simulink model "CementPlantVer1"  (R2019b)
settings: Solver=ode4  StartTime=0.0  StopTime=inf  FixedStep=0.01  RelTol=1e-3
(part 2 of 2)

== system CementPlantVer1/Clinker Fan 2 ==
  Input Frequence : Inport
  Motor Enable : Inport  Port=2
  Constant : Constant  Value=0
  Divide : Product  Inputs=*/
  Frequency Constant : Constant  Value=50
  Frequency Constant FB : Constant  Value=50
  Motor Transfer Function : TransferFcn  Denominator=[1 3.156 1]
  Output coefficient : Constant  Value=1350
  Product : Product
  Product1 : Product
  Saturation : Saturate  UpperLimit=50  LowerLimit=0
  Switch : Switch  Threshold=1
  Output RPM : Outport
  Output Frequence : Outport  Port=2
  wires:
  Product/1 -> Output RPM/1
  Frequency Constant FB/1 -> Product1/2
  Output coefficient/1 -> Product/1
  Frequency Constant/1 -> Divide/2
  Motor Transfer Function/1 -> Product/2, Product1/1
  Input Frequence/1 -> Divide/1
  Saturation/1 -> Output Frequence/1
  Product1/1 -> Saturation/1
  Divide/1 -> Switch/1
  Switch/1 -> Motor Transfer Function/1
  Motor Enable/1 -> Switch/2
  Constant/1 -> Switch/3

== system CementPlantVer1/Clinker Fan 3 ==
  Input Frequence : Inport
  Motor Enable : Inport  Port=2
  Constant : Constant  Value=0
  Divide : Product  Inputs=*/
  Frequency Constant : Constant  Value=50
  Frequency Constant FB : Constant  Value=50
  Motor Transfer Function : TransferFcn  Denominator=[1 3.156 1]
  Output coefficient : Constant  Value=1350
  Product : Product
  Product1 : Product
  Saturation : Saturate  UpperLimit=50  LowerLimit=0
  Switch : Switch  Threshold=1
  Output RPM : Outport
  Output Frequence : Outport  Port=2
  wires:
  Product/1 -> Output RPM/1
  Frequency Constant FB/1 -> Product1/2
  Output coefficient/1 -> Product/1
  Frequency Constant/1 -> Divide/2
  Motor Transfer Function/1 -> Product/2, Product1/1
  Input Frequence/1 -> Divide/1
  Saturation/1 -> Output Frequence/1
  Product1/1 -> Saturation/1
  Divide/1 -> Switch/1
  Switch/1 -> Motor Transfer Function/1
  Motor Enable/1 -> Switch/2
  Constant/1 -> Switch/3

== system CementPlantVer1/Clinker Fan 4 ==
  Input Frequence : Inport
  Motor Enable : Inport  Port=2
  Constant : Constant  Value=0
  Divide : Product  Inputs=*/
  Frequency Constant : Constant  Value=50
  Frequency Constant FB : Constant  Value=50
  Motor Transfer Function : TransferFcn  Denominator=[1 3.156 1]
  Output coefficient : Constant  Value=1350
  Product : Product
  Product1 : Product
  Saturation : Saturate  UpperLimit=50  LowerLimit=0
  Switch : Switch  Threshold=1
  Output RPM : Outport
  Output Frequence : Outport  Port=2
  wires:
  Product/1 -> Output RPM/1
  Frequency Constant FB/1 -> Product1/2
  Output coefficient/1 -> Product/1
  Frequency Constant/1 -> Divide/2
  Motor Transfer Function/1 -> Product/2, Product1/1
  Input Frequence/1 -> Divide/1
  Saturation/1 -> Output Frequence/1
  Product1/1 -> Saturation/1
  Divide/1 -> Switch/1
  Switch/1 -> Motor Transfer Function/1
  Motor Enable/1 -> Switch/2
  Constant/1 -> Switch/3

== system CementPlantVer1/Clinker In Valve 1 ==
  Opening Percent : Inport
  Enable : Inport  Port=2
  Level of Silo : Inport  Port=3
  Constant : Constant  Value=0
  Delay 1s : TransportDelay
  Divide : Product  Inputs=*/
  Maxium Value : Constant  Value=100
  Output Coefficient : Gain  Gain=OutputGain
  Switch : Switch  Threshold=1
  Switch1 : Switch  Criteria=u2 > Threshold
  Transfer Fnc : TransferFcn  Denominator=[20 1]
  Flow : Outport
  wires:
  Transfer Fnc/1 -> Delay 1s/1
  Enable/1 -> Switch/2
  Constant/1 -> Switch/3, Switch1/3
  Opening Percent/1 -> Divide/1
  Divide/1 -> Switch/1
  Maxium Value/1 -> Divide/2
  Output Coefficient/1 -> Flow/1
  Delay 1s/1 -> Output Coefficient/1
  Switch1/1 -> Transfer Fnc/1
  Switch/1 -> Switch1/1
  Level of Silo/1 -> Switch1/2

== system CementPlantVer1/Clinker In Valve 2 ==
  Opening Percent : Inport
  Enable : Inport  Port=2
  Level of Silo : Inport  Port=3
  Constant : Constant  Value=0
  Delay 1s : TransportDelay
  Divide : Product  Inputs=*/
  Maxium Value : Constant  Value=100
  Output Coefficient : Gain  Gain=OutputGain
  Switch : Switch  Threshold=1
  Switch1 : Switch  Criteria=u2 > Threshold
  Transfer Fnc : TransferFcn  Denominator=[20 1]
  Flow : Outport
  wires:
  Transfer Fnc/1 -> Delay 1s/1
  Enable/1 -> Switch/2
  Constant/1 -> Switch/3, Switch1/3
  Opening Percent/1 -> Divide/1
  Divide/1 -> Switch/1
  Maxium Value/1 -> Divide/2
  Output Coefficient/1 -> Flow/1
  Delay 1s/1 -> Output Coefficient/1
  Switch1/1 -> Transfer Fnc/1
  Switch/1 -> Switch1/1
  Level of Silo/1 -> Switch1/2

== system CementPlantVer1/Clinker PreHeater System ==
  RPM In 1 : Inport
  RPM In 2 : Inport  Port=2
  Flow In : Inport  Port=3
  Enable 10 : Constant
  Enable 8 : Constant
  Power supplied to PreHeater 1 : Subsystem
  Power supplied to PreHeater 2 : Subsystem
  PreHeater Flow Transfer Fnc : TransferFcn  Denominator=[0.5 1]
  PreHeater System : Subsystem
  Sum4 : Sum  Inputs=|++
  Temperature : Outport
  Flow out : Outport  Port=2
  wires:
  Enable 8/1 -> Power supplied to PreHeater 1/2(Enable)
  Enable 10/1 -> Power supplied to PreHeater 2/2(Enable)
  Power supplied to PreHeater 1/1(Power Percent) -> Sum4/1
  Sum4/1 -> PreHeater System/1(Power Percent)
  PreHeater System/1(Temperature) -> Temperature/1
  RPM In 2/1 -> Power supplied to PreHeater 2/1(RPM)
  Power supplied to PreHeater 2/1(Power Percent) -> Sum4/2
  RPM In 1/1 -> Power supplied to PreHeater 1/1(RPM)
  Flow In/1 -> PreHeater Flow Transfer Fnc/1
  PreHeater Flow Transfer Fnc/1 -> Flow out/1

== system CementPlantVer1/Clinker Rotary Kiln ==
  RPM In 1 : Inport
  RPM In 2 : Inport  Port=2
  RPM In 3 : Inport  Port=3
  Flow In : Inport  Port=4
  Rotary Kiln Frequence : Inport  Port=5
  Clinker : Subsystem
  Enable 2 : Constant
  Enable 4 : Constant
  Enable 6 : Constant
  Power supplied to Clinker 1 : Subsystem
  Power supplied to Clinker 2 : Subsystem
  Power supplied to Clinker 3 : Subsystem
  Rotary Kiln Motor : Subsystem
  Sum : Sum  Inputs=3
  Temperature : Outport
  Flow Out : Outport  Port=2
  Rotary Kiln RPM : Outport  Port=3
  Rotary Kiln Frequence FB : Outport  Port=4
  wires:
  Sum/1 -> Clinker/1(Power Percent)
  Enable 4/1 -> Power supplied to Clinker 2/2(Enable)
  Enable 2/1 -> Power supplied to Clinker 1/2(Enable)
  Clinker/1(Temperature) -> Temperature/1
  RPM In 3/1 -> Power supplied to Clinker 3/1(RPM)
  Power supplied to Clinker 1/1(Power Percent) -> Sum/1
  Power supplied to Clinker 2/1(Power Percent) -> Sum/2
  Power supplied to Clinker 3/1(Power Percent) -> Sum/3
  Enable 6/1 -> Power supplied to Clinker 3/2(Enable)
  RPM In 2/1 -> Power supplied to Clinker 2/1(RPM)
  RPM In 1/1 -> Power supplied to Clinker 1/1(RPM)
  Flow In/1 -> Rotary Kiln Motor/1(Flow In)
  Rotary Kiln Frequence/1 -> Rotary Kiln Motor/2(Frequence In)
  Rotary Kiln Motor/1(Flow out) -> Flow Out/1
  Rotary Kiln Motor/2(RPM out) -> Rotary Kiln RPM/1
  Rotary Kiln Motor/3(Frequence FB) -> Rotary Kiln Frequence FB/1

== system CementPlantVer1/Clinker Silo 1 ==
  Qin : Inport
  Qout : Inport  Port=2
  A : Gain  Gain=1/(3.14*3*3)
  Convert h to s : Constant  Value=3600
  Density of Clay : Constant  Value=DensityOfMaterial
  Divide : Product  Inputs=*/
  Divide1 : Product  Inputs=*/
  High Operator : RelationalOperator  OutDataTypeStr=boolean  RndMeth=Simplest
  High Level Set (m) : Constant  Value=HighLevelSet
  Low Operator : RelationalOperator  Operator=<=  OutDataTypeStr=boolean  RndMeth=Simplest
  Low Level Set (m) : Constant  Value=LowLevelSet
  Output Coefficient : Gain  Gain=OutputGain
  Saturation Limit : Saturate  UpperLimit=20  LowerLimit=0
  Sum1 : Sum  Inputs=|+-
  Transfer Fnc of Silo : TransferFcn  Denominator=[1 0]
  Level : Outport
  High : Outport  Port=2
  Low : Outport  Port=3
  wires:
  A/1 -> Output Coefficient/1
  Low Operator/1 -> Low/1
  High Level Set (m)/1 -> High Operator/2
  Low Level Set (m)/1 -> Low Operator/2
  Density of Clay/1 -> Divide/2
  Output Coefficient/1 -> Saturation Limit/1
  Convert h to s/1 -> Divide1/2
  Transfer Fnc of Silo/1 -> A/1
  Divide1/1 -> Transfer Fnc of Silo/1
  High Operator/1 -> High/1
  Saturation Limit/1 -> Level/1, Low Operator/1, High Operator/1
  Divide/1 -> Divide1/1
  Sum1/1 -> Divide/1
  Qin/1 -> Sum1/1
  Qout/1 -> Sum1/2

== system CementPlantVer1/Clinker Silo 2 ==
  Qin : Inport
  Qout : Inport  Port=2
  A : Gain  Gain=1/(3.14*3*3)
  Convert h to s : Constant  Value=3600
  Density of Clay : Constant  Value=DensityOfMaterial
  Divide : Product  Inputs=*/
  Divide1 : Product  Inputs=*/
  High Operator : RelationalOperator  OutDataTypeStr=boolean  RndMeth=Simplest
  High Level Set (m) : Constant  Value=HighLevelSet
  Low Operator : RelationalOperator  Operator=<=  OutDataTypeStr=boolean  RndMeth=Simplest
  Low Level Set (m) : Constant  Value=LowLevelSet
  Output Coefficient : Gain  Gain=OutputGain
  Saturation Limit : Saturate  UpperLimit=20  LowerLimit=0
  Sum1 : Sum  Inputs=|+-
  Transfer Fnc of Silo : TransferFcn  Denominator=[1 0]
  Level : Outport
  High : Outport  Port=2
  Low : Outport  Port=3
  wires:
  A/1 -> Output Coefficient/1
  Low Operator/1 -> Low/1
  High Level Set (m)/1 -> High Operator/2
  Low Level Set (m)/1 -> Low Operator/2
  Density of Clay/1 -> Divide/2
  Output Coefficient/1 -> Saturation Limit/1
  Convert h to s/1 -> Divide1/2
  Transfer Fnc of Silo/1 -> A/1
  Divide1/1 -> Transfer Fnc of Silo/1
  High Operator/1 -> High/1
  Saturation Limit/1 -> Level/1, Low Operator/1, High Operator/1
  Divide/1 -> Divide1/1
  Sum1/1 -> Divide/1
  Qin/1 -> Sum1/1
  Qout/1 -> Sum1/2

== system CementPlantVer1/CoalMill Fan 1 ==
  Input Frequence : Inport
  Motor Enable : Inport  Port=2
  Constant : Constant  Value=0
  Divide : Product  Inputs=*/
  Frequency Constant : Constant  Value=50
  Frequency Constant FB : Constant  Value=50
  Motor Transfer Function : TransferFcn  Denominator=[1 3.156 1]
  Output coefficient : Constant  Value=1350
  Product : Product
  Product1 : Product
  Saturation : Saturate  UpperLimit=50  LowerLimit=0
  Switch : Switch  Threshold=1
  Output RPM : Outport
  Output Frequence : Outport  Port=2
  wires:
  Product/1 -> Output RPM/1
  Frequency Constant FB/1 -> Product1/2
  Output coefficient/1 -> Product/1
  Frequency Constant/1 -> Divide/2
  Motor Transfer Function/1 -> Product/2, Product1/1
  Input Frequence/1 -> Divide/1
  Saturation/1 -> Output Frequence/1
  Product1/1 -> Saturation/1
  Divide/1 -> Switch/1
  Switch/1 -> Motor Transfer Function/1
  Motor Enable/1 -> Switch/2
  Constant/1 -> Switch/3

== system CementPlantVer1/CoalMill Pump 1 ==
  Input Frequence : Inport
  Motor Enable : Inport  Port=2
  Constant : Constant  Value=0
  Divide : Product  Inputs=*/
  Frequency Constant : Constant  Value=50
  Frequency Constant FB : Constant  Value=50
  Motor Transfer Function : TransferFcn  Denominator=[1 1.1 1]
  Output coefficient : Constant  Value=1350
  Product : Product
  Product1 : Product
  Saturation : Saturate  UpperLimit=50  LowerLimit=0
  Switch : Switch  Threshold=1
  Output RPM : Outport
  Output Frequence : Outport  Port=2
  wires:
  Product/1 -> Output RPM/1
  Frequency Constant FB/1 -> Product1/2
  Output coefficient/1 -> Product/1
  Frequency Constant/1 -> Divide/2
  Motor Transfer Function/1 -> Product/2, Product1/1
  Input Frequence/1 -> Divide/1
  Saturation/1 -> Output Frequence/1
  Product1/1 -> Saturation/1
  Divide/1 -> Switch/1
  Switch/1 -> Motor Transfer Function/1
  Motor Enable/1 -> Switch/2
  Constant/1 -> Switch/3

== system CementPlantVer1/CoalMill Pump 2 ==
  Input Frequence : Inport
  Motor Enable : Inport  Port=2
  Constant : Constant  Value=0
  Divide : Product  Inputs=*/
  Frequency Constant : Constant  Value=50
  Frequency Constant FB : Constant  Value=50
  Motor Transfer Function : TransferFcn  Denominator=[1 1.1 1]
  Output coefficient : Constant  Value=1350
  Product : Product
  Product1 : Product
  Saturation : Saturate  UpperLimit=50  LowerLimit=0
  Switch : Switch  Threshold=1
  Output RPM : Outport
  Output Frequence : Outport  Port=2
  wires:
  Product/1 -> Output RPM/1
  Frequency Constant FB/1 -> Product1/2
  Output coefficient/1 -> Product/1
  Frequency Constant/1 -> Divide/2
  Motor Transfer Function/1 -> Product/2, Product1/1
  Input Frequence/1 -> Divide/1
  Saturation/1 -> Output Frequence/1
  Product1/1 -> Saturation/1
  Divide/1 -> Switch/1
  Switch/1 -> Motor Transfer Function/1
  Motor Enable/1 -> Switch/2
  Constant/1 -> Switch/3

== system CementPlantVer1/CoalMill Pump 3 ==
  Input Frequence : Inport
  Motor Enable : Inport  Port=2
  Constant : Constant  Value=0
  Divide : Product  Inputs=*/
  Frequency Constant : Constant  Value=50
  Frequency Constant FB : Constant  Value=50
  Motor Transfer Function : TransferFcn  Denominator=[1 1.1 1]
  Output coefficient : Constant  Value=1350
  Product : Product
  Product1 : Product
  Saturation : Saturate  UpperLimit=50  LowerLimit=0
  Switch : Switch  Threshold=1
  Output RPM : Outport
  Output Frequence : Outport  Port=2
  wires:
  Product/1 -> Output RPM/1
  Frequency Constant FB/1 -> Product1/2
  Output coefficient/1 -> Product/1
  Frequency Constant/1 -> Divide/2
  Motor Transfer Function/1 -> Product/2, Product1/1
  Input Frequence/1 -> Divide/1
  Saturation/1 -> Output Frequence/1
  Product1/1 -> Saturation/1
  Divide/1 -> Switch/1
  Switch/1 -> Motor Transfer Function/1
  Motor Enable/1 -> Switch/2
  Constant/1 -> Switch/3

== system CementPlantVer1/CoalMill Pump 4 ==
  Input Frequence : Inport
  Motor Enable : Inport  Port=2
  Constant : Constant  Value=0
  Divide : Product  Inputs=*/
  Frequency Constant : Constant  Value=50
  Frequency Constant FB : Constant  Value=50
  Motor Transfer Function : TransferFcn  Denominator=[1 1.1 1]
  Output coefficient : Constant  Value=1350
  Product : Product
  Product1 : Product
  Saturation : Saturate  UpperLimit=50  LowerLimit=0
  Switch : Switch  Threshold=1
  Output RPM : Outport
  Output Frequence : Outport  Port=2
  wires:
  Product/1 -> Output RPM/1
  Frequency Constant FB/1 -> Product1/2
  Output coefficient/1 -> Product/1
  Frequency Constant/1 -> Divide/2
  Motor Transfer Function/1 -> Product/2, Product1/1
  Input Frequence/1 -> Divide/1
  Saturation/1 -> Output Frequence/1
  Product1/1 -> Saturation/1
  Divide/1 -> Switch/1
  Switch/1 -> Motor Transfer Function/1
  Motor Enable/1 -> Switch/2
  Constant/1 -> Switch/3

== system CementPlantVer1/Gypsum Silo ==
  Qin : Inport
  Qout : Inport  Port=2
  A : Gain  Gain=1/(3.14*3*3)
  Convert h to s : Constant  Value=3600
  Density of Clay : Constant  Value=DensityOfMaterial
  Divide : Product  Inputs=*/
  Divide1 : Product  Inputs=*/
  High Operator : RelationalOperator  OutDataTypeStr=boolean  RndMeth=Simplest
  High Level Set (m) : Constant  Value=HighLevelSet
  Low Operator : RelationalOperator  Operator=<=  OutDataTypeStr=boolean  RndMeth=Simplest
  Low Level Set (m) : Constant  Value=LowLevelSet
  Output Coefficient : Gain  Gain=OutputGain
  Saturation Limit : Saturate  UpperLimit=20  LowerLimit=0
  Sum1 : Sum  Inputs=|+-
  Transfer Fnc of Silo : TransferFcn  Denominator=[1 0]
  Level : Outport
  High : Outport  Port=2
  Low : Outport  Port=3
  wires:
  A/1 -> Output Coefficient/1
  Low Operator/1 -> Low/1
  High Level Set (m)/1 -> High Operator/2
  Low Level Set (m)/1 -> Low Operator/2
  Density of Clay/1 -> Divide/2
  Output Coefficient/1 -> Saturation Limit/1
  Convert h to s/1 -> Divide1/2
  Transfer Fnc of Silo/1 -> A/1
  Divide1/1 -> Transfer Fnc of Silo/1
  High Operator/1 -> High/1
  Saturation Limit/1 -> Level/1, Low Operator/1, High Operator/1
  Divide/1 -> Divide1/1
  Sum1/1 -> Divide/1
  Qin/1 -> Sum1/1
  Qout/1 -> Sum1/2

== system CementPlantVer1/Iron Silo ==
  Qin : Inport
  Qout : Inport  Port=2
  A : Gain  Gain=1/(3.14*3*3)
  Convert h to s : Constant  Value=3600
  Density of Clay : Constant  Value=DensityOfMaterial
  Divide : Product  Inputs=*/
  Divide1 : Product  Inputs=*/
  High Operator : RelationalOperator  OutDataTypeStr=boolean  RndMeth=Simplest
  High Level Set (m) : Constant  Value=HighLevelSet
  Low Operator : RelationalOperator  Operator=<=  OutDataTypeStr=boolean  RndMeth=Simplest
  Low Level Set (m) : Constant  Value=LowLevelSet
  Output Coefficient : Gain  Gain=OutputGain
  Saturation Limit : Saturate  UpperLimit=20  LowerLimit=0
  Sum1 : Sum  Inputs=|+-
  Transfer Fnc of Silo : TransferFcn  Denominator=[1 0]
  Level : Outport
  High : Outport  Port=2
  Low : Outport  Port=3
  wires:
  A/1 -> Output Coefficient/1
  Low Operator/1 -> Low/1
  High Level Set (m)/1 -> High Operator/2
  Low Level Set (m)/1 -> Low Operator/2
  Density of Clay/1 -> Divide/2
  Output Coefficient/1 -> Saturation Limit/1
  Convert h to s/1 -> Divide1/2
  Transfer Fnc of Silo/1 -> A/1
  Divide1/1 -> Transfer Fnc of Silo/1
  High Operator/1 -> High/1
  Saturation Limit/1 -> Level/1, Low Operator/1, High Operator/1
  Divide/1 -> Divide1/1
  Sum1/1 -> Divide/1
  Qin/1 -> Sum1/1
  Qout/1 -> Sum1/2

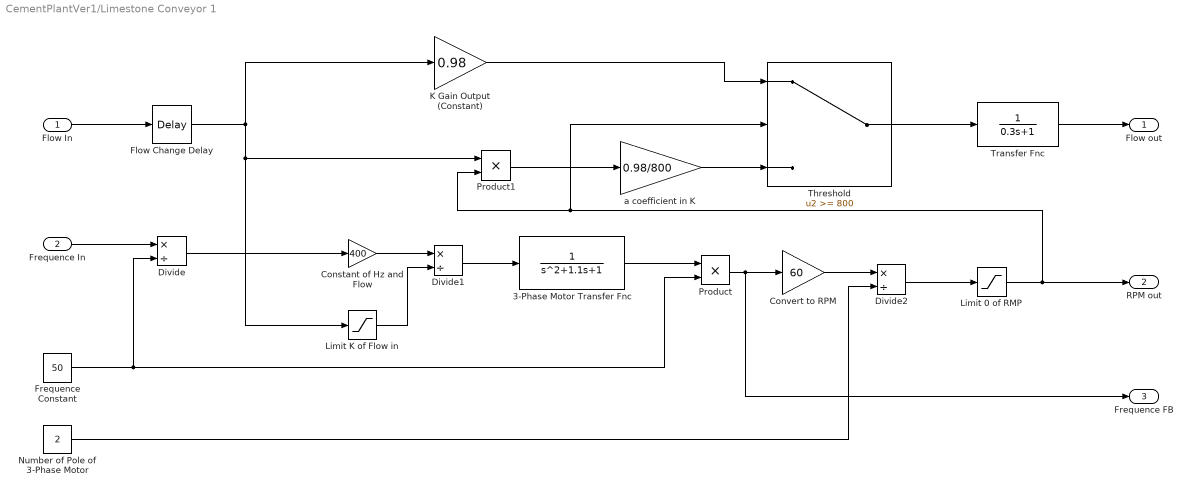
== system CementPlantVer1/Limestone Conveyor 1 ==
  Flow In : Inport
  Frequence In : Inport  Port=2
  3-Phase Motor Transfer Fnc : TransferFcn  Denominator=[1 1.1 1]
  Constant of Hz and Flow : Gain  Gain=400
  Convert to RPM : Gain  Gain=60
  Divide : Product  Inputs=*/
  Divide1 : Product  Inputs=*/
  Divide2 : Product  Inputs=*/
  Flow Change Delay : TransportDelay  DelayTime=0.5
  Frequence Constant : Constant  Value=50
  K Gain Output (Constant) : Gain  Gain=0.98
  Limit 0 of RMP : Saturate  UpperLimit=inf  LowerLimit=0
  Limit K of Flow in : Saturate  UpperLimit=inf  LowerLimit=400
  Number of Pole of 3-Phase Motor : Constant  Value=2
  Product : Product
  Product1 : Product
  Threshold : Switch  Threshold=800
  Transfer Fnc : TransferFcn  Denominator=[0.3 1]
  a coefficient in K : Gain  Gain=0.98/800
  Flow out : Outport
  RPM out : Outport  Port=2
  Frequence FB : Outport  Port=3
  wires:
  Constant of Hz and Flow/1 -> Divide1/1
  Limit K of Flow in/1 -> Divide1/2
  Divide1/1 -> 3-Phase Motor Transfer Fnc/1
  Limit 0 of RMP/1 -> RPM out/1, Threshold/2, Product1/2
  Flow In/1 -> Flow Change Delay/1
  Flow Change Delay/1 -> Product1/1, Limit K of Flow in/1, K Gain Output (Constant)/1
  K Gain Output (Constant)/1 -> Threshold/1
  Frequence In/1 -> Divide/1
  Divide/1 -> Constant of Hz and Flow/1
  Frequence Constant/1 -> Product/2, Divide/2
  3-Phase Motor Transfer Fnc/1 -> Product/1
  Product/1 -> Frequence FB/1, Convert to RPM/1
  Convert to RPM/1 -> Divide2/1
  Divide2/1 -> Limit 0 of RMP/1
  Number of Pole of 3-Phase Motor/1 -> Divide2/2
  Threshold/1 -> Transfer Fnc/1
  Transfer Fnc/1 -> Flow out/1
  Product1/1 -> a coefficient in K/1
  a coefficient in K/1 -> Threshold/3

== system CementPlantVer1/Limestone Conveyor 2 ==
  Flow In : Inport
  Frequence In : Inport  Port=2
  3-Phase Motor Transfer Fnc : TransferFcn  Denominator=[1 1.1 1]
  Constant of Hz and Flow : Gain  Gain=400
  Convert to RPM : Gain  Gain=60
  Divide : Product  Inputs=*/
  Divide1 : Product  Inputs=*/
  Divide2 : Product  Inputs=*/
  Flow Change Delay : TransportDelay  DelayTime=0.5
  Frequence Constant : Constant  Value=50
  K Gain Output (Constant) : Gain  Gain=0.98
  Limit 0 of RMP : Saturate  UpperLimit=inf  LowerLimit=0
  Limit K of Flow in : Saturate  UpperLimit=inf  LowerLimit=400
  Number of Pole of 3-Phase Motor : Constant  Value=2
  Product : Product
  Product1 : Product
  Threshold : Switch  Threshold=800
  Transfer Fnc : TransferFcn  Denominator=[0.3 1]
  a coefficient in K : Gain  Gain=0.98/800
  Flow out : Outport
  RPM out : Outport  Port=2
  Frequence FB : Outport  Port=3
  wires:
  Constant of Hz and Flow/1 -> Divide1/1
  Limit K of Flow in/1 -> Divide1/2
  Divide1/1 -> 3-Phase Motor Transfer Fnc/1
  Limit 0 of RMP/1 -> RPM out/1, Threshold/2, Product1/2
  Flow In/1 -> Flow Change Delay/1
  Flow Change Delay/1 -> Product1/1, Limit K of Flow in/1, K Gain Output (Constant)/1
  K Gain Output (Constant)/1 -> Threshold/1
  Frequence In/1 -> Divide/1
  Divide/1 -> Constant of Hz and Flow/1
  Frequence Constant/1 -> Product/2, Divide/2
  3-Phase Motor Transfer Fnc/1 -> Product/1
  Product/1 -> Frequence FB/1, Convert to RPM/1
  Convert to RPM/1 -> Divide2/1
  Divide2/1 -> Limit 0 of RMP/1
  Number of Pole of 3-Phase Motor/1 -> Divide2/2
  Threshold/1 -> Transfer Fnc/1
  Transfer Fnc/1 -> Flow out/1
  Product1/1 -> a coefficient in K/1
  a coefficient in K/1 -> Threshold/3

== system CementPlantVer1/Limestone Conveyor 3 ==
  Flow In : Inport
  Frequence In : Inport  Port=2
  3-Phase Motor Transfer Fnc : TransferFcn  Denominator=[1 1.1 1]
  Constant of Hz and Flow : Gain  Gain=400
  Convert to RPM : Gain  Gain=60
  Divide : Product  Inputs=*/
  Divide1 : Product  Inputs=*/
  Divide2 : Product  Inputs=*/
  Flow Change Delay : TransportDelay  DelayTime=0.5
  Frequence Constant : Constant  Value=50
  K Gain Output (Constant) : Gain  Gain=0.98
  Limit 0 of RMP : Saturate  UpperLimit=inf  LowerLimit=0
  Limit K of Flow in : Saturate  UpperLimit=inf  LowerLimit=400
  Number of Pole of 3-Phase Motor : Constant  Value=2
  Product : Product
  Product1 : Product
  Threshold : Switch  Threshold=800
  Transfer Fnc : TransferFcn  Denominator=[0.3 1]
  a coefficient in K : Gain  Gain=0.98/800
  Flow out : Outport
  RPM out : Outport  Port=2
  Frequence FB : Outport  Port=3
  wires:
  Constant of Hz and Flow/1 -> Divide1/1
  Limit K of Flow in/1 -> Divide1/2
  Divide1/1 -> 3-Phase Motor Transfer Fnc/1
  Limit 0 of RMP/1 -> RPM out/1, Threshold/2, Product1/2
  Flow In/1 -> Flow Change Delay/1
  Flow Change Delay/1 -> Product1/1, Limit K of Flow in/1, K Gain Output (Constant)/1
  K Gain Output (Constant)/1 -> Threshold/1
  Frequence In/1 -> Divide/1
  Divide/1 -> Constant of Hz and Flow/1
  Frequence Constant/1 -> Product/2, Divide/2
  3-Phase Motor Transfer Fnc/1 -> Product/1
  Product/1 -> Frequence FB/1, Convert to RPM/1
  Convert to RPM/1 -> Divide2/1
  Divide2/1 -> Limit 0 of RMP/1
  Number of Pole of 3-Phase Motor/1 -> Divide2/2
  Threshold/1 -> Transfer Fnc/1
  Transfer Fnc/1 -> Flow out/1
  Product1/1 -> a coefficient in K/1
  a coefficient in K/1 -> Threshold/3

== system CementPlantVer1/Limestone Crusher 1 ==
  Flow In : Inport
  Frequence In : Inport  Port=2
  3-Phase Motor Transfer Fnc : TransferFcn  Denominator=[1 2.5 1]
  Constant of Hz and Flow : Gain  Gain=400
  Convert to RPM : Gain  Gain=60
  Divide : Product  Inputs=*/
  Divide1 : Product  Inputs=*/
  Divide2 : Product  Inputs=*/
  Flow Change Delay : TransportDelay  DelayTime=0.5
  Frequence Constant : Constant  Value=50
  K Gain Output (Constant) : Gain
  Limit 0 of RMP : Saturate  UpperLimit=inf  LowerLimit=0
  Limit K of Flow in : Saturate  UpperLimit=inf  LowerLimit=400
  Number of Pole of 3-Phase Motor : Constant  Value=2
  Product : Product
  Product1 : Product
  Threshold : Switch  Threshold=800
  Transfer Fnc : TransferFcn  Denominator=[0.1 1]
  a coefficient in K : Gain  Gain=1/800
  Flow out : Outport
  Frequence FB : Outport  Port=2
  wires:
  Constant of Hz and Flow/1 -> Divide1/1
  Limit K of Flow in/1 -> Divide1/2
  Divide1/1 -> 3-Phase Motor Transfer Fnc/1
  Limit 0 of RMP/1 -> Threshold/2, Product1/2
  Flow In/1 -> Flow Change Delay/1
  Flow Change Delay/1 -> Product1/1, Limit K of Flow in/1, K Gain Output (Constant)/1
  K Gain Output (Constant)/1 -> Threshold/1
  Frequence In/1 -> Divide/1
  Divide/1 -> Constant of Hz and Flow/1
  Frequence Constant/1 -> Product/2, Divide/2
  3-Phase Motor Transfer Fnc/1 -> Product/1
  Product/1 -> Frequence FB/1, Convert to RPM/1
  Convert to RPM/1 -> Divide2/1
  Divide2/1 -> Limit 0 of RMP/1
  Number of Pole of 3-Phase Motor/1 -> Divide2/2
  Threshold/1 -> Transfer Fnc/1
  Transfer Fnc/1 -> Flow out/1
  Product1/1 -> a coefficient in K/1
  a coefficient in K/1 -> Threshold/3

== system CementPlantVer1/Limestone Crusher 2 ==
  Flow In : Inport
  Frequence In : Inport  Port=2
  3-Phase Motor Transfer Fnc : TransferFcn  Denominator=[1 2.5 1]
  Constant of Hz and Flow : Gain  Gain=400
  Convert to RPM : Gain  Gain=60
  Divide : Product  Inputs=*/
  Divide1 : Product  Inputs=*/
  Divide2 : Product  Inputs=*/
  Flow Change Delay : TransportDelay  DelayTime=0.5
  Frequence Constant : Constant  Value=50
  K Gain Output (Constant) : Gain
  Limit 0 of RMP : Saturate  UpperLimit=inf  LowerLimit=0
  Limit K of Flow in : Saturate  UpperLimit=inf  LowerLimit=400
  Number of Pole of 3-Phase Motor : Constant  Value=2
  Product : Product
  Product1 : Product
  Threshold : Switch  Threshold=800
  Transfer Fnc : TransferFcn  Denominator=[0.1 1]
  a coefficient in K : Gain  Gain=1/800
  Flow out : Outport
  Frequence FB : Outport  Port=2
  wires:
  Constant of Hz and Flow/1 -> Divide1/1
  Limit K of Flow in/1 -> Divide1/2
  Divide1/1 -> 3-Phase Motor Transfer Fnc/1
  Limit 0 of RMP/1 -> Threshold/2, Product1/2
  Flow In/1 -> Flow Change Delay/1
  Flow Change Delay/1 -> Product1/1, Limit K of Flow in/1, K Gain Output (Constant)/1
  K Gain Output (Constant)/1 -> Threshold/1
  Frequence In/1 -> Divide/1
  Divide/1 -> Constant of Hz and Flow/1
  Frequence Constant/1 -> Product/2, Divide/2
  3-Phase Motor Transfer Fnc/1 -> Product/1
  Product/1 -> Frequence FB/1, Convert to RPM/1
  Convert to RPM/1 -> Divide2/1
  Divide2/1 -> Limit 0 of RMP/1
  Number of Pole of 3-Phase Motor/1 -> Divide2/2
  Threshold/1 -> Transfer Fnc/1
  Transfer Fnc/1 -> Flow out/1
  Product1/1 -> a coefficient in K/1
  a coefficient in K/1 -> Threshold/3

== system CementPlantVer1/Limestone Storage ==
  Qin : Inport
  Qout : Inport  Port=2
  A : Gain  Gain=1/(3.14*3*3)
  Convert h to s : Constant  Value=3600
  Density of Clay : Constant  Value=DensityOfMaterial
  Divide : Product  Inputs=*/
  Divide1 : Product  Inputs=*/
  High Operator : RelationalOperator  OutDataTypeStr=boolean  RndMeth=Simplest
  High Level Set (m) : Constant  Value=HighLevelSet
  Low Operator : RelationalOperator  Operator=<=  OutDataTypeStr=boolean  RndMeth=Simplest
  Low Level Set (m) : Constant  Value=LowLevelSet
  Output Coefficient : Gain  Gain=OutputGain
  Saturation Limit : Saturate  UpperLimit=20  LowerLimit=0
  Sum1 : Sum  Inputs=|+-
  Transfer Fnc of Silo : TransferFcn  Denominator=[1 0]
  Level : Outport
  High : Outport  Port=2
  Low : Outport  Port=3
  wires:
  A/1 -> Output Coefficient/1
  Low Operator/1 -> Low/1
  High Level Set (m)/1 -> High Operator/2
  Low Level Set (m)/1 -> Low Operator/2
  Density of Clay/1 -> Divide/2
  Output Coefficient/1 -> Saturation Limit/1
  Convert h to s/1 -> Divide1/2
  Transfer Fnc of Silo/1 -> A/1
  Divide1/1 -> Transfer Fnc of Silo/1
  High Operator/1 -> High/1
  Saturation Limit/1 -> Level/1, Low Operator/1, High Operator/1
  Divide/1 -> Divide1/1
  Sum1/1 -> Divide/1
  Qin/1 -> Sum1/1
  Qout/1 -> Sum1/2

== system CementPlantVer1/Limestone Valve 1 ==
  Opening Percent : Inport
  Enable : Inport  Port=2
  Level of Silo : Inport  Port=3
  Constant : Constant  Value=0
  Delay 1s : TransportDelay
  Divide : Product  Inputs=*/
  Maxium Value : Constant  Value=100
  Output Coefficient : Gain  Gain=OutputGain
  Switch : Switch  Threshold=1
  Switch1 : Switch  Criteria=u2 > Threshold
  Transfer Fnc : TransferFcn  Denominator=[20 1]
  Flow : Outport
  wires:
  Transfer Fnc/1 -> Delay 1s/1
  Enable/1 -> Switch/2
  Constant/1 -> Switch/3, Switch1/3
  Opening Percent/1 -> Divide/1
  Divide/1 -> Switch/1
  Maxium Value/1 -> Divide/2
  Output Coefficient/1 -> Flow/1
  Delay 1s/1 -> Output Coefficient/1
  Switch1/1 -> Transfer Fnc/1
  Switch/1 -> Switch1/1
  Level of Silo/1 -> Switch1/2

== system CementPlantVer1/RawMill Conveyor 1 ==
  Input Frequence : Inport
  Enable : Inport  Port=2
  3-Phase Motor Transfer Fnc : TransferFcn  Denominator=[1 1 1]
  Constant : Constant  Value=0
  Divide : Product  Inputs=*/
  Frequence Coefficient : Gain  Gain=50
  Maxium Value : Constant  Value=50
  Output Coefficient : Gain  Gain=OutputGain
  Switch : Switch  Threshold=1
  Flow : Outport
  FeedBack Frequence : Outport  Port=2
  wires:
  3-Phase Motor Transfer Fnc/1 -> Frequence Coefficient/1, Output Coefficient/1
  Output Coefficient/1 -> Flow/1
  Switch/1 -> 3-Phase Motor Transfer Fnc/1
  Enable/1 -> Switch/2
  Constant/1 -> Switch/3
  Input Frequence/1 -> Divide/1
  Divide/1 -> Switch/1
  Maxium Value/1 -> Divide/2
  Frequence Coefficient/1 -> FeedBack Frequence/1

== system CementPlantVer1/RawMill Conveyor 2 ==
  Input Frequence : Inport
  Enable : Inport  Port=2
  3-Phase Motor Transfer Fnc : TransferFcn  Denominator=[1 1 1]
  Constant : Constant  Value=0
  Divide : Product  Inputs=*/
  Frequence Coefficient : Gain  Gain=50
  Maxium Value : Constant  Value=50
  Output Coefficient : Gain  Gain=OutputGain
  Switch : Switch  Threshold=1
  Flow : Outport
  FeedBack Frequence : Outport  Port=2
  wires:
  3-Phase Motor Transfer Fnc/1 -> Frequence Coefficient/1, Output Coefficient/1
  Output Coefficient/1 -> Flow/1
  Switch/1 -> 3-Phase Motor Transfer Fnc/1
  Enable/1 -> Switch/2
  Constant/1 -> Switch/3
  Input Frequence/1 -> Divide/1
  Divide/1 -> Switch/1
  Maxium Value/1 -> Divide/2
  Frequence Coefficient/1 -> FeedBack Frequence/1

== system CementPlantVer1/RawMill Conveyor 3 ==
  Flow In : Inport
  Frequence In : Inport  Port=2
  3-Phase Motor Transfer Fnc : TransferFcn  Denominator=[1 1.1 1]
  Constant of Hz and Flow : Gain  Gain=400
  Convert to RPM : Gain  Gain=60
  Divide : Product  Inputs=*/
  Divide1 : Product  Inputs=*/
  Divide2 : Product  Inputs=*/
  Flow Change Delay : TransportDelay  DelayTime=0.5
  Frequence Constant : Constant  Value=50
  K Gain Output (Constant) : Gain  Gain=0.98
  Limit 0 of RMP : Saturate  UpperLimit=inf  LowerLimit=0
  Limit K of Flow in : Saturate  UpperLimit=inf  LowerLimit=400
  Number of Pole of 3-Phase Motor : Constant  Value=2
  Product : Product
  Product1 : Product
  Threshold : Switch  Threshold=800
  Transfer Fnc : TransferFcn  Denominator=[0.3 1]
  a coefficient in K : Gain  Gain=0.98/800
  Flow out : Outport
  RPM out : Outport  Port=2
  Frequence FB : Outport  Port=3
  wires:
  Constant of Hz and Flow/1 -> Divide1/1
  Limit K of Flow in/1 -> Divide1/2
  Divide1/1 -> 3-Phase Motor Transfer Fnc/1
  Limit 0 of RMP/1 -> RPM out/1, Threshold/2, Product1/2
  Flow In/1 -> Flow Change Delay/1
  Flow Change Delay/1 -> Product1/1, Limit K of Flow in/1, K Gain Output (Constant)/1
  K Gain Output (Constant)/1 -> Threshold/1
  Frequence In/1 -> Divide/1
  Divide/1 -> Constant of Hz and Flow/1
  Frequence Constant/1 -> Product/2, Divide/2
  3-Phase Motor Transfer Fnc/1 -> Product/1
  Product/1 -> Frequence FB/1, Convert to RPM/1
  Convert to RPM/1 -> Divide2/1
  Divide2/1 -> Limit 0 of RMP/1
  Number of Pole of 3-Phase Motor/1 -> Divide2/2
  Threshold/1 -> Transfer Fnc/1
  Transfer Fnc/1 -> Flow out/1
  Product1/1 -> a coefficient in K/1
  a coefficient in K/1 -> Threshold/3

== system CementPlantVer1/RawMill Conveyor 4 ==
  Flow In : Inport
  Frequence In : Inport  Port=2
  3-Phase Motor Transfer Fnc : TransferFcn  Denominator=[1 1.1 1]
  Constant of Hz and Flow : Gain  Gain=400
  Convert to RPM : Gain  Gain=60
  Divide : Product  Inputs=*/
  Divide1 : Product  Inputs=*/
  Divide2 : Product  Inputs=*/
  Flow Change Delay : TransportDelay  DelayTime=0.5
  Frequence Constant : Constant  Value=50
  K Gain Output (Constant) : Gain  Gain=0.98
  Limit 0 of RMP : Saturate  UpperLimit=inf  LowerLimit=0
  Limit K of Flow in : Saturate  UpperLimit=inf  LowerLimit=400
  Number of Pole of 3-Phase Motor : Constant  Value=2
  Product : Product
  Product1 : Product
  Threshold : Switch  Threshold=800
  Transfer Fnc : TransferFcn  Denominator=[0.3 1]
  a coefficient in K : Gain  Gain=0.98/800
  Flow out : Outport
  RPM out : Outport  Port=2
  Frequence FB : Outport  Port=3
  wires:
  Constant of Hz and Flow/1 -> Divide1/1
  Limit K of Flow in/1 -> Divide1/2
  Divide1/1 -> 3-Phase Motor Transfer Fnc/1
  Limit 0 of RMP/1 -> RPM out/1, Threshold/2, Product1/2
  Flow In/1 -> Flow Change Delay/1
  Flow Change Delay/1 -> Product1/1, Limit K of Flow in/1, K Gain Output (Constant)/1
  K Gain Output (Constant)/1 -> Threshold/1
  Frequence In/1 -> Divide/1
  Divide/1 -> Constant of Hz and Flow/1
  Frequence Constant/1 -> Product/2, Divide/2
  3-Phase Motor Transfer Fnc/1 -> Product/1
  Product/1 -> Frequence FB/1, Convert to RPM/1
  Convert to RPM/1 -> Divide2/1
  Divide2/1 -> Limit 0 of RMP/1
  Number of Pole of 3-Phase Motor/1 -> Divide2/2
  Threshold/1 -> Transfer Fnc/1
  Transfer Fnc/1 -> Flow out/1
  Product1/1 -> a coefficient in K/1
  a coefficient in K/1 -> Threshold/3

== system CementPlantVer1/RawMill Conveyor 5 ==
  Flow In : Inport
  Frequence In : Inport  Port=2
  3-Phase Motor Transfer Fnc : TransferFcn  Denominator=[1 1.1 1]
  Constant of Hz and Flow : Gain  Gain=400
  Convert to RPM : Gain  Gain=60
  Divide : Product  Inputs=*/
  Divide1 : Product  Inputs=*/
  Divide2 : Product  Inputs=*/
  Flow Change Delay : TransportDelay  DelayTime=0.5
  Frequence Constant : Constant  Value=50
  K Gain Output (Constant) : Gain  Gain=0.98
  Limit 0 of RMP : Saturate  UpperLimit=inf  LowerLimit=0
  Limit K of Flow in : Saturate  UpperLimit=inf  LowerLimit=400
  Number of Pole of 3-Phase Motor : Constant  Value=2
  Product : Product
  Product1 : Product
  Threshold : Switch  Threshold=800
  Transfer Fnc : TransferFcn  Denominator=[0.3 1]
  a coefficient in K : Gain  Gain=0.98/800
  Flow out : Outport
  RPM out : Outport  Port=2
  Frequence FB : Outport  Port=3
  wires:
  Constant of Hz and Flow/1 -> Divide1/1
  Limit K of Flow in/1 -> Divide1/2
  Divide1/1 -> 3-Phase Motor Transfer Fnc/1
  Limit 0 of RMP/1 -> RPM out/1, Threshold/2, Product1/2
  Flow In/1 -> Flow Change Delay/1
  Flow Change Delay/1 -> Product1/1, Limit K of Flow in/1, K Gain Output (Constant)/1
  K Gain Output (Constant)/1 -> Threshold/1
  Frequence In/1 -> Divide/1
  Divide/1 -> Constant of Hz and Flow/1
  Frequence Constant/1 -> Product/2, Divide/2
  3-Phase Motor Transfer Fnc/1 -> Product/1
  Product/1 -> Frequence FB/1, Convert to RPM/1
  Convert to RPM/1 -> Divide2/1
  Divide2/1 -> Limit 0 of RMP/1
  Number of Pole of 3-Phase Motor/1 -> Divide2/2
  Threshold/1 -> Transfer Fnc/1
  Transfer Fnc/1 -> Flow out/1
  Product1/1 -> a coefficient in K/1
  a coefficient in K/1 -> Threshold/3

== system CementPlantVer1/RawMill Iron Valve In ==
  Open/Close : Inport
  Constant : Constant  Value=0
  Constant1 : Constant  Value=FlowConstant
  Switch : Switch  Threshold=1
  Transfer Fcn : TransferFcn  Denominator=[0.5 1]
  Flow Out : Outport
  wires:
  Open/Close/1 -> Switch/2
  Constant/1 -> Switch/3
  Constant1/1 -> Switch/1
  Switch/1 -> Transfer Fcn/1
  Transfer Fcn/1 -> Flow Out/1

== system CementPlantVer1/RawMill Iron Valve Out ==
  Opening Percent : Inport
  Enable : Inport  Port=2
  Level of Silo : Inport  Port=3
  Constant : Constant  Value=0
  Delay 1s : TransportDelay
  Divide : Product  Inputs=*/
  Maxium Value : Constant  Value=100
  Output Coefficient : Gain  Gain=OutputGain
  Switch : Switch  Threshold=1
  Switch1 : Switch  Criteria=u2 > Threshold
  Transfer Fnc : TransferFcn  Denominator=[20 1]
  Flow : Outport
  wires:
  Transfer Fnc/1 -> Delay 1s/1
  Enable/1 -> Switch/2
  Constant/1 -> Switch/3, Switch1/3
  Opening Percent/1 -> Divide/1
  Divide/1 -> Switch/1
  Maxium Value/1 -> Divide/2
  Output Coefficient/1 -> Flow/1
  Delay 1s/1 -> Output Coefficient/1
  Switch1/1 -> Transfer Fnc/1
  Switch/1 -> Switch1/1
  Level of Silo/1 -> Switch1/2

== system CementPlantVer1/RawMill Sand Valve In ==
  Open/Close : Inport
  Constant : Constant  Value=0
  Constant1 : Constant  Value=FlowConstant
  Switch : Switch  Threshold=1
  Transfer Fcn : TransferFcn  Denominator=[0.5 1]
  Flow Out : Outport
  wires:
  Open/Close/1 -> Switch/2
  Constant/1 -> Switch/3
  Constant1/1 -> Switch/1
  Switch/1 -> Transfer Fcn/1
  Transfer Fcn/1 -> Flow Out/1

== system CementPlantVer1/RawMill Sand Valve Out ==
  Opening Percent : Inport
  Enable : Inport  Port=2
  Level of Silo : Inport  Port=3
  Constant : Constant  Value=0
  Delay 1s : TransportDelay
  Divide : Product  Inputs=*/
  Maxium Value : Constant  Value=100
  Output Coefficient : Gain  Gain=OutputGain
  Switch : Switch  Threshold=1
  Switch1 : Switch  Criteria=u2 > Threshold
  Transfer Fnc : TransferFcn  Denominator=[20 1]
  Flow : Outport
  wires:
  Transfer Fnc/1 -> Delay 1s/1
  Enable/1 -> Switch/2
  Constant/1 -> Switch/3, Switch1/3
  Opening Percent/1 -> Divide/1
  Divide/1 -> Switch/1
  Maxium Value/1 -> Divide/2
  Output Coefficient/1 -> Flow/1
  Delay 1s/1 -> Output Coefficient/1
  Switch1/1 -> Transfer Fnc/1
  Switch/1 -> Switch1/1
  Level of Silo/1 -> Switch1/2

== system CementPlantVer1/RawMill Silo 1 ==
  Qin : Inport
  Qout : Inport  Port=2
  A : Gain  Gain=1/(3.14*3*3)
  Convert h to s : Constant  Value=3600
  Density of Clay : Constant  Value=DensityOfMaterial
  Divide : Product  Inputs=*/
  Divide1 : Product  Inputs=*/
  High Operator : RelationalOperator  OutDataTypeStr=boolean  RndMeth=Simplest
  High Level Set (m) : Constant  Value=HighLevelSet
  Low Operator : RelationalOperator  Operator=<=  OutDataTypeStr=boolean  RndMeth=Simplest
  Low Level Set (m) : Constant  Value=LowLevelSet
  Output Coefficient : Gain  Gain=OutputGain
  Saturation Limit : Saturate  UpperLimit=20  LowerLimit=0
  Sum1 : Sum  Inputs=|+-
  Transfer Fnc of Silo : TransferFcn  Denominator=[1 0]
  Level : Outport
  High : Outport  Port=2
  Low : Outport  Port=3
  wires:
  A/1 -> Output Coefficient/1
  Low Operator/1 -> Low/1
  High Level Set (m)/1 -> High Operator/2
  Low Level Set (m)/1 -> Low Operator/2
  Density of Clay/1 -> Divide/2
  Output Coefficient/1 -> Saturation Limit/1
  Convert h to s/1 -> Divide1/2
  Transfer Fnc of Silo/1 -> A/1
  Divide1/1 -> Transfer Fnc of Silo/1
  High Operator/1 -> High/1
  Saturation Limit/1 -> Level/1, Low Operator/1, High Operator/1
  Divide/1 -> Divide1/1
  Sum1/1 -> Divide/1
  Qin/1 -> Sum1/1
  Qout/1 -> Sum1/2

== system CementPlantVer1/RawMill Silo 2 ==
  Qin : Inport
  Qout : Inport  Port=2
  A : Gain  Gain=1/(3.14*3*3)
  Convert h to s : Constant  Value=3600
  Density of Clay : Constant  Value=DensityOfMaterial
  Divide : Product  Inputs=*/
  Divide1 : Product  Inputs=*/
  High Operator : RelationalOperator  OutDataTypeStr=boolean  RndMeth=Simplest
  High Level Set (m) : Constant  Value=HighLevelSet
  Low Operator : RelationalOperator  Operator=<=  OutDataTypeStr=boolean  RndMeth=Simplest
  Low Level Set (m) : Constant  Value=LowLevelSet
  Output Coefficient : Gain  Gain=OutputGain
  Saturation Limit : Saturate  UpperLimit=20  LowerLimit=0
  Sum1 : Sum  Inputs=|+-
  Transfer Fnc of Silo : TransferFcn  Denominator=[1 0]
  Level : Outport
  High : Outport  Port=2
  Low : Outport  Port=3
  wires:
  A/1 -> Output Coefficient/1
  Low Operator/1 -> Low/1
  High Level Set (m)/1 -> High Operator/2
  Low Level Set (m)/1 -> Low Operator/2
  Density of Clay/1 -> Divide/2
  Output Coefficient/1 -> Saturation Limit/1
  Convert h to s/1 -> Divide1/2
  Transfer Fnc of Silo/1 -> A/1
  Divide1/1 -> Transfer Fnc of Silo/1
  High Operator/1 -> High/1
  Saturation Limit/1 -> Level/1, Low Operator/1, High Operator/1
  Divide/1 -> Divide1/1
  Sum1/1 -> Divide/1
  Qin/1 -> Sum1/1
  Qout/1 -> Sum1/2

== system CementPlantVer1/Roller Mill 1 ==
  Flow In : Inport
  Frequence In : Inport  Port=2
  3-Phase Motor Transfer Fnc : TransferFcn  Denominator=[1 1.56 1]
  Constant of Hz and Flow : Gain  Gain=400
  Convert to RPM : Gain  Gain=60
  Divide : Product  Inputs=*/
  Divide1 : Product  Inputs=*/
  Divide2 : Product  Inputs=*/
  Flow Change Delay : TransportDelay  DelayTime=0.5
  Frequence Constant : Constant  Value=50
  K Gain Output (Constant) : Gain  Gain=0.8
  Limit 0 of RMP : Saturate  UpperLimit=inf  LowerLimit=0
  Limit K of Flow in : Saturate  UpperLimit=inf  LowerLimit=400
  Number of Pole of 3-Phase Motor : Constant  Value=2
  Product : Product
  Product1 : Product
  Threshold : Switch  Threshold=800
  Transfer Fnc : TransferFcn  Denominator=[0.5 1]
  a coefficient in K : Gain  Gain=0.8/800
  Flow out : Outport
  RPM Out : Outport  Port=2
  Frequence FB : Outport  Port=3
  wires:
  Constant of Hz and Flow/1 -> Divide1/1
  Limit K of Flow in/1 -> Divide1/2
  Divide1/1 -> 3-Phase Motor Transfer Fnc/1
  Limit 0 of RMP/1 -> RPM Out/1, Threshold/2, Product1/2
  Flow In/1 -> Flow Change Delay/1
  Flow Change Delay/1 -> Product1/1, Limit K of Flow in/1, K Gain Output (Constant)/1
  K Gain Output (Constant)/1 -> Threshold/1
  Frequence In/1 -> Divide/1
  Divide/1 -> Constant of Hz and Flow/1
  Frequence Constant/1 -> Product/2, Divide/2
  3-Phase Motor Transfer Fnc/1 -> Product/1
  Product/1 -> Frequence FB/1, Convert to RPM/1
  Convert to RPM/1 -> Divide2/1
  Divide2/1 -> Limit 0 of RMP/1
  Number of Pole of 3-Phase Motor/1 -> Divide2/2
  Threshold/1 -> Transfer Fnc/1
  Transfer Fnc/1 -> Flow out/1
  Product1/1 -> a coefficient in K/1
  a coefficient in K/1 -> Threshold/3

== system CementPlantVer1/Sand Silo ==
  Qin : Inport
  Qout : Inport  Port=2
  A : Gain  Gain=1/(3.14*3*3)
  Convert h to s : Constant  Value=3600
  Density of Clay : Constant  Value=DensityOfMaterial
  Divide : Product  Inputs=*/
  Divide1 : Product  Inputs=*/
  High Operator : RelationalOperator  OutDataTypeStr=boolean  RndMeth=Simplest
  High Level Set (m) : Constant  Value=HighLevelSet
  Low Operator : RelationalOperator  Operator=<=  OutDataTypeStr=boolean  RndMeth=Simplest
  Low Level Set (m) : Constant  Value=LowLevelSet
  Output Coefficient : Gain  Gain=OutputGain
  Saturation Limit : Saturate  UpperLimit=20  LowerLimit=0
  Sum1 : Sum  Inputs=|+-
  Transfer Fnc of Silo : TransferFcn  Denominator=[1 0]
  Level : Outport
  High : Outport  Port=2
  Low : Outport  Port=3
  wires:
  A/1 -> Output Coefficient/1
  Low Operator/1 -> Low/1
  High Level Set (m)/1 -> High Operator/2
  Low Level Set (m)/1 -> Low Operator/2
  Density of Clay/1 -> Divide/2
  Output Coefficient/1 -> Saturation Limit/1
  Convert h to s/1 -> Divide1/2
  Transfer Fnc of Silo/1 -> A/1
  Divide1/1 -> Transfer Fnc of Silo/1
  High Operator/1 -> High/1
  Saturation Limit/1 -> Level/1, Low Operator/1, High Operator/1
  Divide/1 -> Divide1/1
  Sum1/1 -> Divide/1
  Qin/1 -> Sum1/1
  Qout/1 -> Sum1/2

== system CementPlantVer1/Clinker PreHeater System/Power supplied to PreHeater 1 ==
  RPM : Inport
  Enable : Inport  Port=2
  Constant : Constant  Value=0
  Delay 2s : TransportDelay  DelayTime=2
  Divide : Product  Inputs=*/
  Maxium Value : Constant  Value=1350
  Output Coefficient : Gain  Gain=0.7
  Switch : Switch  Threshold=1
  Transfer Fnc : TransferFcn  Denominator=[4 1]
  Power Percent : Outport
  wires:
  Transfer Fnc/1 -> Delay 2s/1
  Delay 2s/1 -> Output Coefficient/1
  Output Coefficient/1 -> Power Percent/1
  Switch/1 -> Transfer Fnc/1
  Enable/1 -> Switch/2
  Constant/1 -> Switch/3
  RPM/1 -> Divide/1
  Divide/1 -> Switch/1
  Maxium Value/1 -> Divide/2

== system CementPlantVer1/Clinker PreHeater System/Power supplied to PreHeater 2 ==
  RPM : Inport
  Enable : Inport  Port=2
  Constant : Constant  Value=0
  Delay 2s : TransportDelay  DelayTime=2
  Divide : Product  Inputs=*/
  Maxium Value : Constant  Value=1350
  Output Coefficient : Gain  Gain=0.3
  Switch : Switch  Threshold=1
  Transfer Fnc : TransferFcn  Denominator=[4 1]
  Power Percent : Outport
  wires:
  Transfer Fnc/1 -> Delay 2s/1
  Delay 2s/1 -> Output Coefficient/1
  Output Coefficient/1 -> Power Percent/1
  Switch/1 -> Transfer Fnc/1
  Enable/1 -> Switch/2
  Constant/1 -> Switch/3
  RPM/1 -> Divide/1
  Divide/1 -> Switch/1
  Maxium Value/1 -> Divide/2

== system CementPlantVer1/Clinker PreHeater System/PreHeater System ==
  Power Percent : Inport
  Delay 20s : TransportDelay  DelayTime=12  BufferSize=2048
  Output Coefficient : Gain
  Transfer Fcn : TransferFcn  Numerator=[900]  Denominator=[15 1]
  Temperature : Outport
  wires:
  Delay 20s/1 -> Output Coefficient/1
  Output Coefficient/1 -> Temperature/1
  Transfer Fcn/1 -> Delay 20s/1
  Power Percent/1 -> Transfer Fcn/1

== system CementPlantVer1/Clinker Rotary Kiln/Clinker ==
  Power Percent : Inport
  Delay 20s : TransportDelay  DelayTime=20  BufferSize=2048
  Output Coefficient : Gain
  Transfer Fcn : TransferFcn  Numerator=[1450]  Denominator=[30 1]
  Temperature : Outport
  wires:
  Delay 20s/1 -> Output Coefficient/1
  Output Coefficient/1 -> Temperature/1
  Transfer Fcn/1 -> Delay 20s/1
  Power Percent/1 -> Transfer Fcn/1

== system CementPlantVer1/Clinker Rotary Kiln/Power supplied to Clinker 1 ==
  RPM : Inport
  Enable : Inport  Port=2
  Constant : Constant  Value=0
  Delay 2s : TransportDelay  DelayTime=2
  Divide : Product  Inputs=*/
  Maxium Value : Constant  Value=1350
  Output Coefficient : Gain  Gain=0.5
  Switch : Switch  Threshold=1
  Transfer Fnc : TransferFcn  Denominator=[4 1]
  Power Percent : Outport
  wires:
  Transfer Fnc/1 -> Delay 2s/1
  Delay 2s/1 -> Output Coefficient/1
  Output Coefficient/1 -> Power Percent/1
  Switch/1 -> Transfer Fnc/1
  Enable/1 -> Switch/2
  Constant/1 -> Switch/3
  RPM/1 -> Divide/1
  Divide/1 -> Switch/1
  Maxium Value/1 -> Divide/2

== system CementPlantVer1/Clinker Rotary Kiln/Power supplied to Clinker 2 ==
  RPM : Inport
  Enable : Inport  Port=2
  Constant : Constant  Value=0
  Delay 2s : TransportDelay  DelayTime=2
  Divide : Product  Inputs=*/
  Maxium Value : Constant  Value=1350
  Output Coefficient : Gain  Gain=0.5
  Switch : Switch  Threshold=1
  Transfer Fnc : TransferFcn  Denominator=[4 1]
  Power Percent : Outport
  wires:
  Transfer Fnc/1 -> Delay 2s/1
  Delay 2s/1 -> Output Coefficient/1
  Output Coefficient/1 -> Power Percent/1
  Switch/1 -> Transfer Fnc/1
  Enable/1 -> Switch/2
  Constant/1 -> Switch/3
  RPM/1 -> Divide/1
  Divide/1 -> Switch/1
  Maxium Value/1 -> Divide/2

== system CementPlantVer1/Clinker Rotary Kiln/Power supplied to Clinker 3 ==
  RPM : Inport
  Enable : Inport  Port=2
  Constant : Constant  Value=0
  Delay 2s : TransportDelay  DelayTime=2
  Divide : Product  Inputs=*/
  Maxium Value : Constant  Value=1350
  Output Coefficient : Gain  Gain=0.5
  Switch : Switch  Threshold=1
  Transfer Fnc : TransferFcn  Denominator=[4 1]
  Power Percent : Outport
  wires:
  Transfer Fnc/1 -> Delay 2s/1
  Delay 2s/1 -> Output Coefficient/1
  Output Coefficient/1 -> Power Percent/1
  Switch/1 -> Transfer Fnc/1
  Enable/1 -> Switch/2
  Constant/1 -> Switch/3
  RPM/1 -> Divide/1
  Divide/1 -> Switch/1
  Maxium Value/1 -> Divide/2

== system CementPlantVer1/Clinker Rotary Kiln/Rotary Kiln Motor ==
  Flow In : Inport
  Frequence In : Inport  Port=2
  3-Phase Motor Transfer Fnc : TransferFcn  Denominator=[1 1.1 1]
  Constant of Hz and Flow : Gain  Gain=400
  Convert to RPM : Gain  Gain=60
  Divide : Product  Inputs=*/
  Divide1 : Product  Inputs=*/
  Divide2 : Product  Inputs=*/
  Flow Change Delay : TransportDelay  DelayTime=0.5
  Frequence Constant : Constant  Value=50
  K Gain Output (Constant) : Gain
  Limit 0 of RMP : Saturate  UpperLimit=inf  LowerLimit=0
  Limit K of Flow in : Saturate  UpperLimit=inf  LowerLimit=400
  Number of Pole of 3-Phase Motor : Constant  Value=2
  Product : Product
  Product1 : Product
  Threshold : Switch  Threshold=800
  Transfer Fnc : TransferFcn  Denominator=[0.3 1]
  a coefficient in K : Gain  Gain=1/800
  Flow out : Outport
  RPM out : Outport  Port=2
  Frequence FB : Outport  Port=3
  wires:
  Constant of Hz and Flow/1 -> Divide1/1
  Limit K of Flow in/1 -> Divide1/2
  Divide1/1 -> 3-Phase Motor Transfer Fnc/1
  Limit 0 of RMP/1 -> RPM out/1, Threshold/2, Product1/2
  Flow In/1 -> Flow Change Delay/1
  Flow Change Delay/1 -> Product1/1, Limit K of Flow in/1, K Gain Output (Constant)/1
  K Gain Output (Constant)/1 -> Threshold/1
  Frequence In/1 -> Divide/1
  Divide/1 -> Constant of Hz and Flow/1
  Frequence Constant/1 -> Product/2, Divide/2
  3-Phase Motor Transfer Fnc/1 -> Product/1
  Product/1 -> Frequence FB/1, Convert to RPM/1
  Convert to RPM/1 -> Divide2/1
  Divide2/1 -> Limit 0 of RMP/1
  Number of Pole of 3-Phase Motor/1 -> Divide2/2
  Threshold/1 -> Transfer Fnc/1
  Transfer Fnc/1 -> Flow out/1
  Product1/1 -> a coefficient in K/1
  a coefficient in K/1 -> Threshold/3
